simulink model "trygit_2"  (R2020b)
settings: Solver=VariableStepAuto  StartTime=0.0  StopTime=10.0  RelTol=1e-3
settings Model: Creator=GURU  LastModifiedBy=GURU

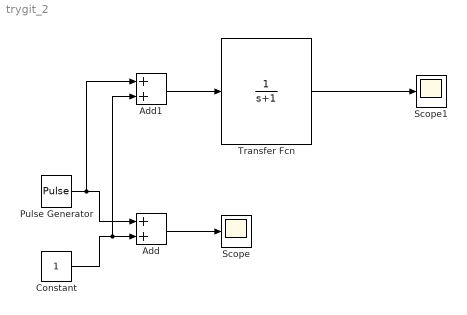
== system trygit_2 ==
  Add : Sum
  Add1 : Sum
  Constant : Constant
  Pulse Generator : DiscretePulseGenerator  PulseType=Time based  Period=10  PulseWidth=5
  Scope : Scope
  Scope1 : Scope
  Transfer Fcn : TransferFcn  Denominator=[1 1]
  wires:
  Pulse Generator/1 -> Add1/1, Add/1
  Constant/1 -> Add1/2, Add/2
  Add/1 -> Scope/1
  Add1/1 -> Transfer Fcn/1
  Transfer Fcn/1 -> Scope1/1
